simulink model "cstr2_control_loops"  (R2019a)
settings: Solver=ode15s  StartTime=0.0  StopTime=10  RelTol=1e-3
values from neighbouring files (symbols this model uses):
  cstr2_const =     [matlab.mat]    (also in prepare_sim.m = struct(); withnmpc.mat)
settings Model: Creator=User  LastModifiedBy=User
settings DebuggingCC: PregeneratedLibrarySubsystemCodeDiagnostic=none  ArithmeticOperatorsInVariantConditions=warning
settings CodeAppCC: StateflowObjectComments=on

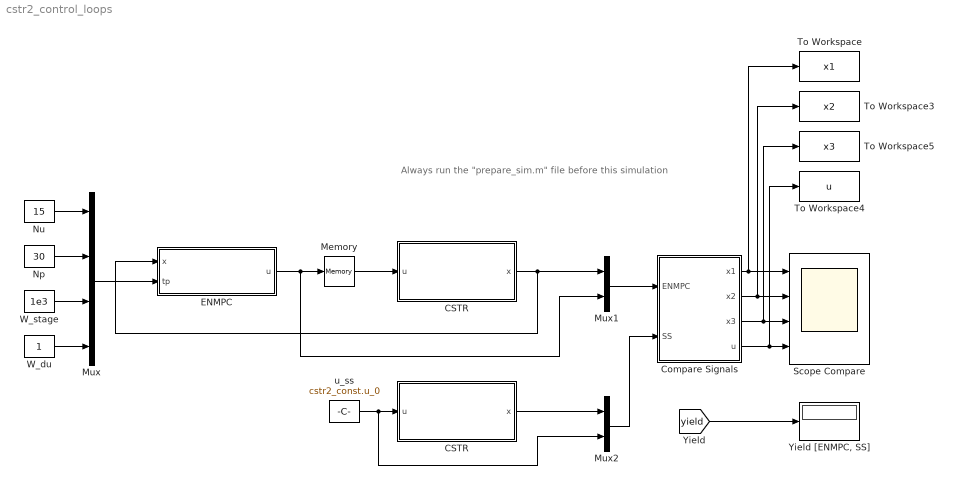
== system cstr2_control_loops ==
  note: Always run the "prepare_sim.m" file before this simulation
  " CSTR " : Subsystem
  " Yield [ENMPC, SS]" : Display
  CSTR : Subsystem
  Compare Signals : Subsystem
  ENMPC : Subsystem
  Memory : Memory  InitialCondition=cstr2_const.u_0
  Mux : Mux
  Mux1 : Mux  Inputs=2
  Mux2 : Mux  Inputs=2
  Np : Constant  Value=30
  Nu : Constant  Value=15
  Scope Compare : Scope  NumInputPorts=4
  To Workspace : ToWorkspace  VariableName=x1  SaveFormat=Structure With Time  SampleTime=-1
  To Workspace3 : ToWorkspace  VariableName=x2  SaveFormat=Structure With Time  SampleTime=-1
  To Workspace4 : ToWorkspace  VariableName=u  SaveFormat=Structure With Time  SampleTime=-1
  To Workspace5 : ToWorkspace  VariableName=x3  SaveFormat=Structure With Time  SampleTime=-1
  W_du : Constant
  W_stage : Constant  Value=1e3
  u_ss : Constant  Value=cstr2_const.u_0
  wires:
  CSTR/1(x) -> Mux1/1, ENMPC/1(x)
  Nu/1 -> Mux/1
  Np/1 -> Mux/2
  W_stage/1 -> Mux/3
  Mux/1 -> ENMPC/2(tp)
  W_du/1 -> Mux/4
  Memory/1 -> CSTR/1(u)
  Mux1/1 -> Compare Signals/1(ENMPC)
  ENMPC/1(u) -> Mux1/2, Memory/1
  u_ss/1 -> " CSTR "/1(u), Mux2/2
  " CSTR "/1(x) -> Mux2/1
  Mux2/1 -> Compare Signals/2(SS)
  [yield] -> " Yield [ENMPC, SS]"/1
  Compare Signals/4(u) -> To Workspace4/1, Scope Compare/4
  Compare Signals/2(x2) -> To Workspace3/1, Scope Compare/2
  Compare Signals/1(x1) -> Scope Compare/1, To Workspace/1
  Compare Signals/3(x3) -> To Workspace5/1, Scope Compare/3

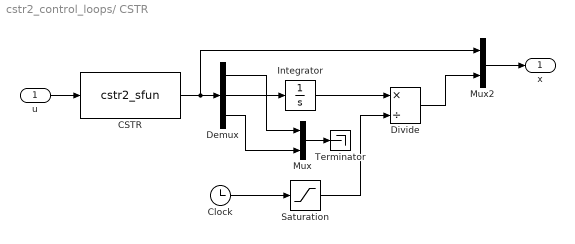
== system cstr2_control_loops/ CSTR  ==
  u : Inport
  CSTR : S-Function  FunctionName=cstr2_sfun  SFunctionDeploymentMode=off  EnableBusSupport=off
  Clock : Clock
  Demux : Demux  Outputs=3
  Divide : Product  Inputs=*/
  Integrator : Integrator
  Mux : Mux  Inputs=2
  Mux2 : Mux  Inputs=2
  Saturation : Saturate  UpperLimit=inf  LowerLimit=cstr2_const.ts
  Terminator : Terminator
  x : Outport
  wires:
  Integrator/1 -> Divide/1
  Divide/1 -> Mux2/2
  CSTR/1 -> Mux2/1, Demux/1
  u/1 -> CSTR/1
  Mux2/1 -> x/1
  Demux/2 -> Integrator/1
  Demux/1 -> Mux/1
  Demux/3 -> Mux/2
  Mux/1 -> Terminator/1
  Clock/1 -> Saturation/1
  Saturation/1 -> Divide/2

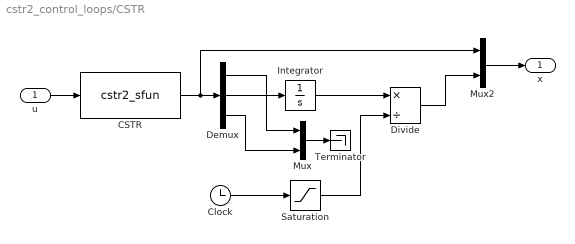
== system cstr2_control_loops/CSTR ==
  u : Inport
  CSTR : S-Function  FunctionName=cstr2_sfun  SFunctionDeploymentMode=off  EnableBusSupport=off
  Clock : Clock
  Demux : Demux  Outputs=3
  Divide : Product  Inputs=*/
  Integrator : Integrator
  Mux : Mux  Inputs=2
  Mux2 : Mux  Inputs=2
  Saturation : Saturate  UpperLimit=inf  LowerLimit=cstr2_const.ts
  Terminator : Terminator
  x : Outport
  wires:
  Integrator/1 -> Divide/1
  Divide/1 -> Mux2/2
  CSTR/1 -> Mux2/1, Demux/1
  u/1 -> CSTR/1
  Mux2/1 -> x/1
  Demux/2 -> Integrator/1
  Demux/1 -> Mux/1
  Demux/3 -> Mux/2
  Mux/1 -> Terminator/1
  Clock/1 -> Saturation/1
  Saturation/1 -> Divide/2

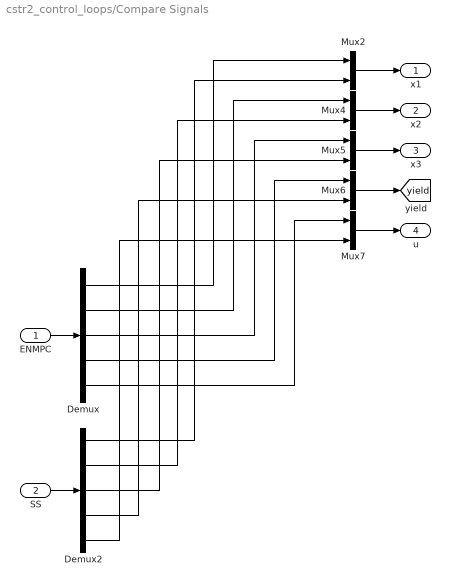
== system cstr2_control_loops/Compare Signals ==
  ENMPC : Inport
  SS : Inport  Port=2
  Demux : Demux  Outputs=5
  Demux2 : Demux  Outputs=5
  Mux{2,4..7} (5 alike) : Mux  Inputs=2
  x1 : Outport
  x2 : Outport  Port=2
  x3 : Outport  Port=3
  u : Outport  Port=4
  tag scope: yield=global
  wires:
  ENMPC/1 -> Demux/1
  Demux/2 -> Mux4/1
  Demux/1 -> Mux2/1
  SS/1 -> Demux2/1
  Demux2/1 -> Mux2/2
  Demux2/2 -> Mux4/2
  Demux/3 -> Mux5/1
  Demux2/3 -> Mux5/2
  Demux/4 -> Mux6/1
  Demux2/4 -> Mux6/2
  Demux/5 -> Mux7/1
  Demux2/5 -> Mux7/2
  Mux6/1 -> [yield]
  Mux5/1 -> x3/1
  Mux4/1 -> x2/1
  Mux2/1 -> x1/1
  Mux7/1 -> u/1

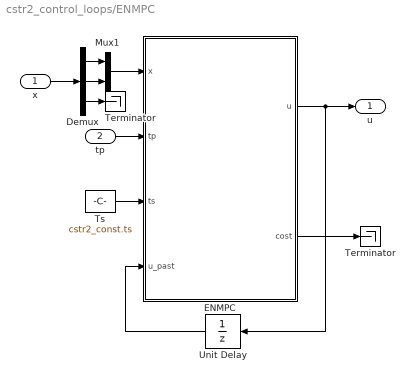
== system cstr2_control_loops/ENMPC ==
  x : Inport
  tp : Inport  Port=2
  Demux : Demux  Outputs=3
  "ENMPC " : MATLAB Function  TreatAsAtomicUnit=on  SystemSampleTime=cstr2_const.ts
  Mux1 : Mux  Inputs=2
  Terminator : Terminator
  "Terminator " : Terminator
  Ts : Constant  Value=cstr2_const.ts
  Unit Delay : UnitDelay  InitialCondition=cstr2_const.u_0  SampleTime=cstr2_const.ts  HasFrameUpgradeWarning=on
  u : Outport
  wires:
  "ENMPC "/1(u) -> u/1, Unit Delay/1
  Unit Delay/1 -> "ENMPC "/4(u_past)
  x/1 -> Demux/1
  tp/1 -> "ENMPC "/2(tp)
  Ts/1 -> "ENMPC "/3(ts)
  "ENMPC "/2(cost) -> "Terminator "/1
  Demux/1 -> Mux1/1
  Demux/2 -> Mux1/2
  Mux1/1 -> "ENMPC "/1(x)
  Demux/3 -> Terminator/1

== matlab function cstr2_control_loops/ENMPC/ENMPC  ==
  data: u output size=[1,1]; cost output size=[1,1]; x input; tp input; ts input; u_past input
function [u, cost] = enmpc(x,tp,ts,u_past)
    u = u_past; cost = 0;
    coder.extrinsic('get_control_input');
    [u,cost] = get_control_input(x,u_past,tp,1,ts);
end
